simulink model "rldepositos"  (R2024a)
settings: Solver=FixedStepDiscrete  StartTime=0.0  StopTime=inf  FixedStep=Ts  RelTol=1e-3  EnableMultiTasking=on
undefined symbols (not defined in the file): DiscIntNeverNeededParam, Q11, Q22, Q33, Q44, R11, R22
libraries: simulink x4, rllib x1
settings Model: Creator=The MathWorks, Inc.  LastModifiedBy=Iván MG
settings SolverCC: AlgebraicLoopSolver=TrustRegion
settings DataIOCC: LimitDataPoints=on  SaveFormat=Array  SignalLoggingName=logsOut
settings OptimizationCC: ReuseModelBlockBuffer=off  ExpressionDepthLimit=2147483647  InitFltsAndDblsToZero=on  LifeSpan=inf
settings DebuggingCC: SaveWithParameterizedLinksMsg=none  UnderspecifiedInitializationDetection=Classic  MergeDetectMultiDrivingBlocksExec=none  SignalResolutionControl=TryResolveAllWithWarning  MultiTaskDSMMsg=warning  FcnCallInpInsideContextMsg=warning  UnconnectedInputMsg=warning  UnconnectedOutputMsg=warning  UnconnectedLineMsg=warning  AllowSymbolicDim=off  StateNameClashWarn=warning  SFUnexpectedBacktrackingDiag=warning  SFNoUnconditionalDefaultTransitionDiag=warning  SFExecutionAtInitializationDiag=none  ArithmeticOperatorsInVariantConditions=warning
settings HardwareCC: ProdBitPerPointer=32  ProdBitPerSizeT=32  ProdBitPerPtrDiffT=32  ProdLargestAtomicFloat=None  ProdIntDivRoundTo=Undefined  ProdEndianess=Unspecified  ProdWordSize=32  ProdHWDeviceType=Specified
settings ModelReferenceCC: EnableRefExpFcnMdlSchedulingChecks=on  PropagateSignalLabelsOutOfModel=off
settings SFSimCC: SimUseLocalCustomCode=off  CustomCodeUndefinedFunction=UseInterfaceOnly
settings RTWCC: RTWUseLocalCustomCode=off  GPUComputeCapability=3.5  DLArmComputeVersion=19.05
settings CodeAppCC: StateflowObjectComments=on
settings GRTTargetCC: TargetFcnLib=ansi_tfl_tmw.mat  TargetLangStandard=C89/C90 (ANSI)  CombineOutputUpdateFcns=off  GRTInterface=on
settings ConfigComp: CovMetricSettings=dw  CovSaveCumulativeToWorkspaceVar=on  CovSaveSingleToWorkspaceVar=on  CovExternalEMLEnable=off

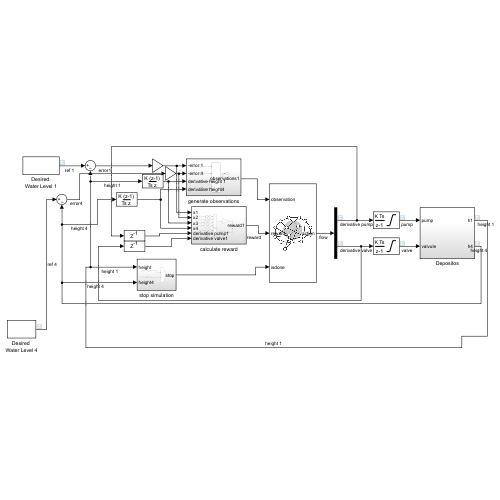
[thumbnail: Simulink's stored preview of the top-level diagram]
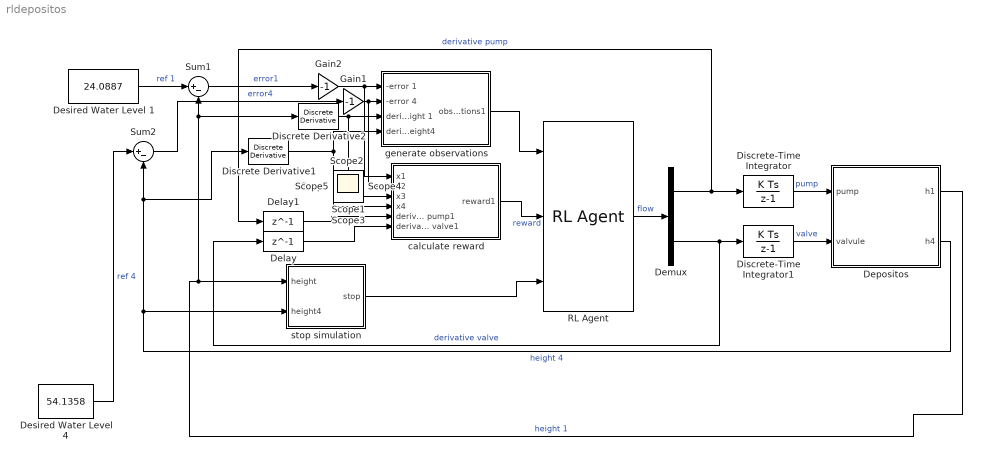
== system rldepositos ==
  Delay : Delay  DelayLength=1  InitialCondition=0
  Delay1 : Delay  DelayLength=1  InitialCondition=0
  Demux : Demux  Outputs=2
  Depositos : Subsystem
  Desired Water Level 1 : Constant  Value=24.0887
  Desired Water Level 4 : Constant  Value=54.1358
  Discrete Derivative1 : simulink/Discrete/Discrete Derivative  gainval=1.0  ICPrevScaledInput=0.0  OutMin=[]  OutMax=[]  OutDataType=fixdt(1, 16)  OutScaling=2^-10  DoSatur=off
  Discrete Derivative2 : simulink/Discrete/Discrete Derivative  gainval=1.0  ICPrevScaledInput=0.0  OutMin=[]  OutMax=[]  OutDataType=fixdt(1, 16)  OutScaling=2^-10  DoSatur=off
  Discrete-Time Integrator : DiscreteIntegrator  SampleTime=-1  LimitOutput=on  UpperSaturationLimit=100  LowerSaturationLimit=0  ICPrevOutput=DiscIntNeverNeededParam  ICPrevScaledInput=DiscIntNeverNeededParam
  Discrete-Time Integrator1 : DiscreteIntegrator  SampleTime=-1  LimitOutput=on  UpperSaturationLimit=100  LowerSaturationLimit=0  ICPrevOutput=DiscIntNeverNeededParam  ICPrevScaledInput=DiscIntNeverNeededParam
  Gain1 : Gain  Gain=-1
  Gain2 : Gain  Gain=-1
  RL Agent : rllib/RL Agent  Agent=agent  ExternalActionAsInput=off  ProvideLastAction=off  ProvideCumRwd=off  TreatAsDirectFeedthrough=on  UseStrictObservationDataTypes=off
  Sum1 : Sum  Inputs=|+-  SaturateOnIntegerOverflow=on
  Sum2 : Sum  Inputs=|+-  SaturateOnIntegerOverflow=on
  calculate reward : Subsystem
  generate observations : Subsystem
  stop simulation : Subsystem
  Scope{,1..5} (6 alike) : Scope
  wires:
  Desired Water Level 1/1 -> Sum1/1  "ref 1"
  Depositos/1(h1) -> Discrete Derivative2/1, Sum1/2, stop simulation/1(height)  "height 1"
  stop simulation/1(stop) -> RL Agent/3
  calculate reward/1(reward1) -> RL Agent/2  "reward"
  generate observations/1(observations1) -> RL Agent/1
  Depositos/2(h4) -> stop simulation/2(height4), Discrete Derivative1/1, Sum2/2  "height 4"
  Desired Water Level 4/1 -> Sum2/1  "ref 4"
  RL Agent/1 -> Demux/1  "flow"
  Gain1/1 -> calculate reward/2(x2), generate observations/2(-error 4)
  Gain2/1 -> calculate reward/1(x1), generate observations/1(-error 1)
  Sum1/1 -> Gain2/1  "error1"
  Sum2/1 -> Gain1/1  "error4"
  Discrete Derivative2/1 -> calculate reward/3(x3), generate observations/3(derivative height 1)
  Discrete Derivative1/1 -> generate observations/4(derivative height4), calculate reward/4(x4)
  Discrete-Time Integrator/1 -> Depositos/1(pump)  "pump"
  Discrete-Time Integrator1/1 -> Depositos/2(valvule)  "valve"
  Demux/2 -> Delay/1, Discrete-Time Integrator1/1  "derivative valve"
  Demux/1 -> Delay1/1, Discrete-Time Integrator/1  "derivative pump"
  Delay/1 -> calculate reward/6(derivative valve1)
  Delay1/1 -> calculate reward/5(derivative pump1)

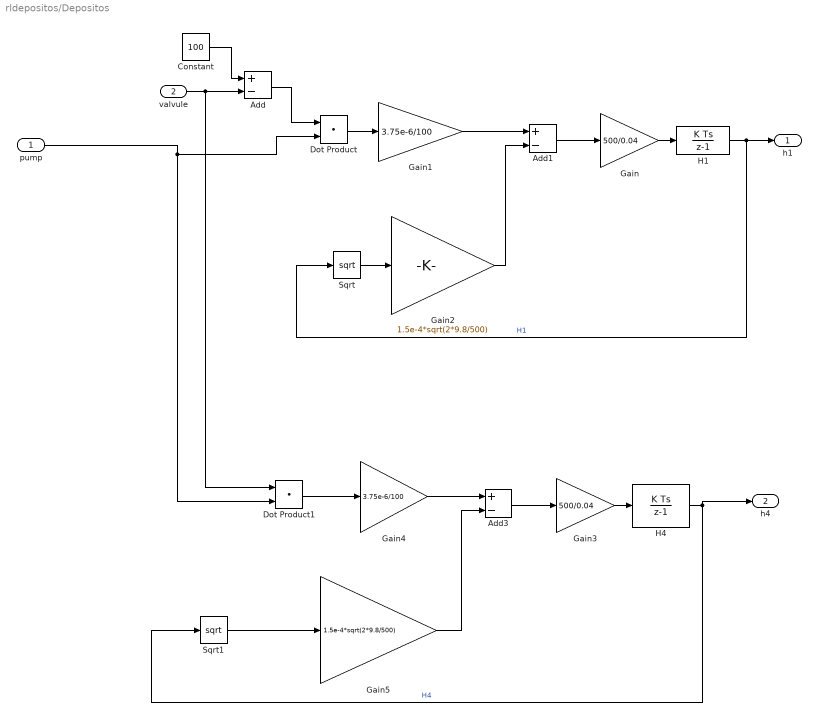
== system rldepositos/Depositos ==
  pump : Inport
  valvule : Inport  Port=2
  Add : Sum  Inputs=+-
  Add1 : Sum  Inputs=+-
  Add3 : Sum  Inputs=+-
  Constant : Constant  Value=100
  Dot Product : DotProduct  OutDataTypeStr=Inherit: Inherit via internal rule
  Dot Product1 : DotProduct  OutDataTypeStr=Inherit: Inherit via internal rule
  Gain : Gain  Gain=500/0.04
  Gain1 : Gain  Gain=3.75e-6/100
  Gain2 : Gain  Gain=1.5e-4*sqrt(2*9.8/500)
  Gain3 : Gain  Gain=500/0.04
  Gain4 : Gain  Gain=3.75e-6/100
  Gain5 : Gain  Gain=1.5e-4*sqrt(2*9.8/500)
  H1 : DiscreteIntegrator  SampleTime=-1  LimitOutput=on  UpperSaturationLimit=100  LowerSaturationLimit=0  ICPrevOutput=DiscIntNeverNeededParam  ICPrevScaledInput=DiscIntNeverNeededParam
  H4 : DiscreteIntegrator  SampleTime=-1  LimitOutput=on  UpperSaturationLimit=100  LowerSaturationLimit=0  ICPrevOutput=DiscIntNeverNeededParam  ICPrevScaledInput=DiscIntNeverNeededParam
  Sqrt : Sqrt
  Sqrt1 : Sqrt
  h1 : Outport
  h4 : Outport  Port=2
  wires:
  Gain1/1 -> Add1/1
  Sqrt1/1 -> Gain5/1
  Dot Product1/1 -> Gain4/1
  Gain/1 -> H1/1
  Add3/1 -> Gain3/1
  Gain2/1 -> Add1/2
  Gain3/1 -> H4/1
  valvule/1 -> Dot Product1/1, Add/2
  pump/1 -> Dot Product1/2, Dot Product/2
  Gain4/1 -> Add3/1
  Gain5/1 -> Add3/2
  Dot Product/1 -> Gain1/1
  Sqrt/1 -> Gain2/1
  Add1/1 -> Gain/1
  H4/1 -> Sqrt1/1, h4/1  "H4"
  Add/1 -> Dot Product/1
  Constant/1 -> Add/1
  H1/1 -> h1/1, Sqrt/1  "H1"

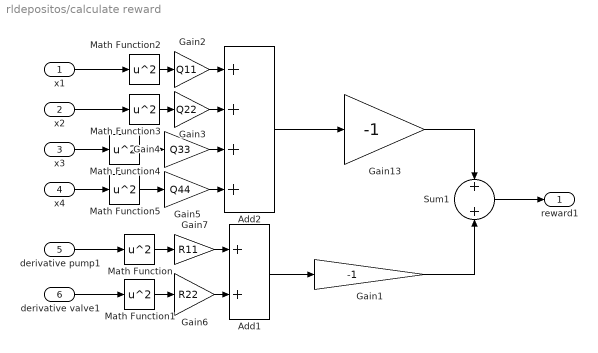
== system rldepositos/calculate reward ==
  x1 : Inport
  x2 : Inport  Port=2
  x3 : Inport  Port=3
  x4 : Inport  Port=4
  derivative pump1 : Inport  Port=5
  derivative valve1 : Inport  Port=6
  Add1 : Sum
  Add2 : Sum  Inputs=++++
  Gain1 : Gain  Gain=-1
  Gain13 : Gain  Gain=-1
  Gain2 : Gain  Gain=Q11
  Gain3 : Gain  Gain=Q22
  Gain4 : Gain  Gain=Q33
  Gain5 : Gain  Gain=Q44
  Gain6 : Gain  Gain=R22
  Gain7 : Gain  Gain=R11
  Math Function{,1..5} (6 alike) : Math  Operator=square
  Sum1 : Sum  OutDataTypeStr=double
  reward1 : Outport  VectorParamsAs1DForOutWhenUnconnected=off
  wires:
  Add2/1 -> Gain13/1
  Gain13/1 -> Sum1/1
  Sum1/1 -> reward1/1
  derivative pump1/1 -> Math Function/1
  derivative valve1/1 -> Math Function1/1
  Add1/1 -> Gain1/1
  x1/1 -> Math Function2/1
  Math Function3/1 -> Gain3/1
  Gain1/1 -> Sum1/2
  x2/1 -> Math Function3/1
  x4/1 -> Math Function5/1
  Math Function5/1 -> Gain5/1
  x3/1 -> Math Function4/1
  Math Function2/1 -> Gain2/1
  Gain2/1 -> Add2/1
  Gain3/1 -> Add2/2
  Gain4/1 -> Add2/3
  Math Function4/1 -> Gain4/1
  Gain5/1 -> Add2/4
  Math Function1/1 -> Gain6/1
  Gain6/1 -> Add1/2
  Math Function/1 -> Gain7/1
  Gain7/1 -> Add1/1

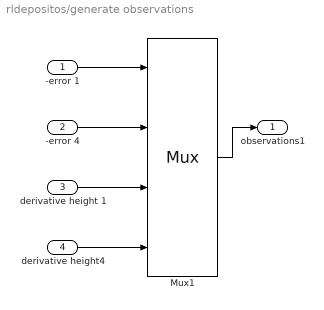
== system rldepositos/generate observations ==
  -error 1 : Inport
  -error 4 : Inport  Port=2
  derivative height 1 : Inport  Port=3
  derivative height4 : Inport  Port=4
  Mux1 : Mux
  observations1 : Outport  VectorParamsAs1DForOutWhenUnconnected=off
  wires:
  derivative height 1/1 -> Mux1/3
  Mux1/1 -> observations1/1
  -error 4/1 -> Mux1/2
  -error 1/1 -> Mux1/1
  derivative height4/1 -> Mux1/4

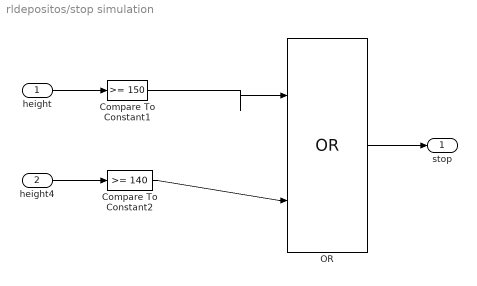
== system rldepositos/stop simulation ==
  height : Inport
  height4 : Inport  Port=2
  Compare To Constant1 : simulink/Logic and Bit Operations/Compare To Constant  relop=>=  const=150  OutDataTypeStr=boolean
  Compare To Constant2 : simulink/Logic and Bit Operations/Compare To Constant  relop=>=  const=140  OutDataTypeStr=boolean
  OR : Logic  Operator=OR  IconShape=distinctive  AllPortsSameDT=off  OutDataTypeStr=boolean
  stop : Outport  VectorParamsAs1DForOutWhenUnconnected=off
  wires:
  height/1 -> Compare To Constant1/1
  Compare To Constant1/1 -> OR/1
  OR/1 -> stop/1
  height4/1 -> Compare To Constant2/1
  Compare To Constant2/1 -> OR/2
